simulink model "controllo_LQ_infinito_tc_LMI"  (R2021a)
settings: Solver=VariableStepAuto  StartTime=0.0  StopTime=tsim  RelTol=1e-3
values from neighbouring files (symbols this model uses):
  b = 20    [main.m]
  c = 718    [main.m]
  F_lmi_tc = double(K)*inv(double(Y))    [main.m]
  f_w = 0    [main.m]
  g = 9.81    [main.m]
  k = 2.5    [main.m]
  m = 500    [main.m]
  p_a = 1.184    [main.m]
  theta_a = 298    [main.m]
  u_eq = k*(theta - theta_a)    (= 199.411134904)    [main.m]
  V = 2000    [main.m]
  x_0 = [550;0;150]    [main.m]
  x_eq = [600;0;theta]    [main.m]
settings Model: Creator=Randy  LastModifiedBy=Randy

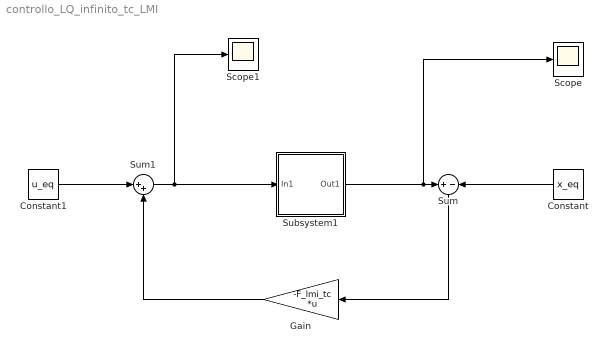
== system controllo_LQ_infinito_tc_LMI ==
  Constant : Constant  Value=x_eq
  Constant1 : Constant  Value=u_eq
  Gain : Gain  Gain=-F_lmi_tc  Multiplication=Matrix(K*u)
  Scope : Scope
  Scope1 : Scope
  Subsystem1 : Subsystem
  Sum : Sum  Inputs=+|-
  Sum1 : Sum  Inputs=|++
  wires:
  Sum/1 -> Gain/1
  Constant/1 -> Sum/2
  Gain/1 -> Sum1/2
  Sum1/1 -> Scope1/1, Subsystem1/1(In1)
  Constant1/1 -> Sum1/1
  Subsystem1/1(Out1) -> Scope/1, Sum/1

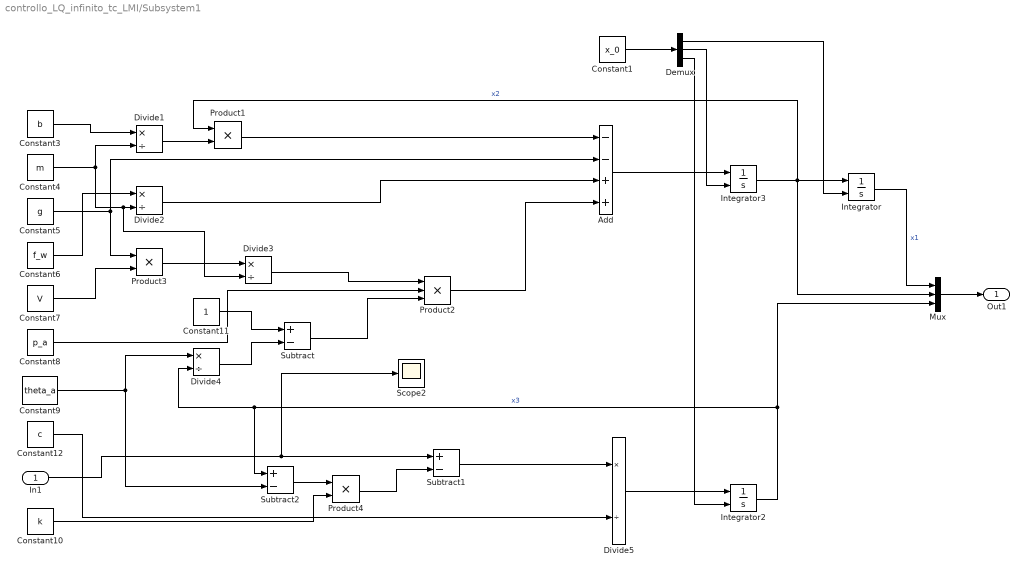
== system controllo_LQ_infinito_tc_LMI/Subsystem1 ==
  In1 : Inport
  Add : Sum  Inputs=--++
  Constant1 : Constant  Value=x_0
  Constant10 : Constant  Value=k
  Constant11 : Constant
  Constant12 : Constant  Value=c
  Constant3 : Constant  Value=b
  Constant4 : Constant  Value=m
  Constant5 : Constant  Value=g
  Constant6 : Constant  Value=f_w
  Constant7 : Constant  Value=V
  Constant8 : Constant  Value=p_a
  Constant9 : Constant  Value=theta_a
  Demux : Demux  Outputs=3
  Divide{1..5} (5 alike) : Product  Inputs=*/
  Integrator : Integrator  InitialConditionSource=external  InitialCondition=680
  Integrator2 : Integrator  InitialConditionSource=external  InitialCondition=200
  Integrator3 : Integrator  InitialConditionSource=external
  Mux : Mux  Inputs=3
  Product1 : Product
  Product2 : Product  Inputs=3
  Product3 : Product
  Product4 : Product
  Scope2 : Scope
  Subtract : Sum  Inputs=+-
  Subtract1 : Sum  Inputs=+-
  Subtract2 : Sum  Inputs=+-
  Out1 : Outport
  wires:
  Integrator2/1 -> Mux/3, Divide4/2, Subtract2/1  "x3"
  Subtract1/1 -> Divide5/1
  Constant6/1 -> Divide2/1
  Constant12/1 -> Divide5/2
  Divide5/1 -> Integrator2/1
  Constant8/1 -> Product2/2
  Add/1 -> Integrator3/1
  Mux/1 -> Out1/1
  Divide3/1 -> Product2/1
  Product1/1 -> Add/1
  Product3/1 -> Divide3/1
  Constant4/1 -> Divide1/2, Divide2/2, Divide3/2
  Integrator/1 -> Mux/1  "x1"
  Divide2/1 -> Add/3
  Integrator3/1 -> Product1/1, Integrator/1, Mux/2  "x2"
  Constant11/1 -> Subtract/1
  Product4/1 -> Subtract1/2
  Constant3/1 -> Divide1/1
  Divide1/1 -> Product1/2
  Subtract2/1 -> Product4/1
  Product2/1 -> Add/4
  Constant7/1 -> Product3/2
  Constant10/1 -> Product4/2
  Divide4/1 -> Subtract/2
  Constant5/1 -> Add/2, Product3/1
  Constant9/1 -> Divide4/1, Subtract2/2
  In1/1 -> Subtract1/1, Scope2/1
  Subtract/1 -> Product2/3
  Constant1/1 -> Demux/1
  Demux/1 -> Integrator/2
  Demux/2 -> Integrator3/2
  Demux/3 -> Integrator2/2
